simulink model "chap1_11"  (R2016a)
settings: Solver=ode5  StartTime=0.0  StopTime=1  FixedStep=0.001  RelTol=1e-3
settings Model: Creator=admin  LastModifiedBy=admin

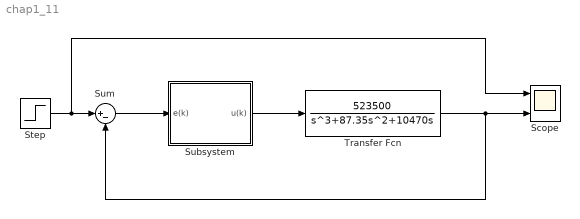
== system chap1_11 ==
  Scope : Scope  NumInputPorts=2
  Step : Step  Time=0  SampleTime=0
  Subsystem : Subsystem  mask{Kp=0.5, Ki=0.001, Kd=0.001, T=0.001, U_m=10}
      mask prompts: Kp "Proportional Kp"; Ki "Integrator Ki"; Kd "Derivative Kd"; T "Sampling period T"; U_m "limit"
      mask Display: disp('Discrete PID')
  Sum : Sum  Inputs=|+-
  Transfer Fcn : TransferFcn  Numerator=[523500]  Denominator=[1 87.35 10470 0]
  wires:
  Step/1 -> Scope/1, Sum/1
  Sum/1 -> Subsystem/1(e(k))
  Subsystem/1("u(k) ") -> Transfer Fcn/1
  Transfer Fcn/1 -> Scope/2, Sum/2

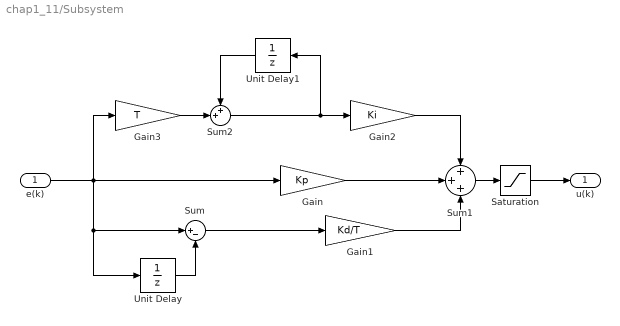
== system chap1_11/Subsystem ==
  e(k) : Inport
  Gain : Gain  Gain=Kp
  Gain1 : Gain  Gain=Kd/T
  Gain2 : Gain  Gain=Ki
  Gain3 : Gain  Gain=T
  Saturation : Saturate  UpperLimit=U_m  LowerLimit=-U_m
  Sum : Sum  Inputs=|+-
  Sum1 : Sum  Inputs=+++
  Sum2 : Sum  Inputs=++|
  Unit Delay : UnitDelay  SampleTime=-1
  Unit Delay1 : UnitDelay  SampleTime=-1
  "u(k) " : Outport
  wires:
  Sum/1 -> Gain1/1
  Unit Delay1/1 -> Sum2/1
  Sum2/1 -> Unit Delay1/1, Gain2/1
  Gain3/1 -> Sum2/2
  Gain1/1 -> Sum1/3
  Saturation/1 -> "u(k) "/1
  e(k)/1 -> Gain3/1, Gain/1, Sum/1, Unit Delay/1
  Sum1/1 -> Saturation/1
  Unit Delay/1 -> Sum/2
  Gain/1 -> Sum1/2
  Gain2/1 -> Sum1/1
